simulink model "untitled1"  (R2024b)
settings: Solver=VariableStepAuto  StartTime=0.0  StopTime=10  RelTol=1e-3
values from neighbouring files (symbols this model uses):
  Cd = [0 1]    [mpc3.m]
  Cr = 87342    [mpc3.m]    (also in prueba_mpc.m; prueba_mpc2.m)
  m = 1400    [mpc3.m]    (also in prueba_mpc.m; prueba_mpc2.m)
  R = 1    [prueba_mpc.m]    (also in prueba_mpc2.m)
  vx = 10    [mpc3.m]    (also in prueba_mpc.m; prueba_mpc2.m)
undefined symbols (not defined in the file or in its folder): Af, F_max, FN, g, mode, mu1, mu2, mu3, theta
libraries: slpidlib x1
settings Model: Creator=inaki  LastModifiedBy=inaki
settings DebuggingCC: AlgebraicLoopMsg=none

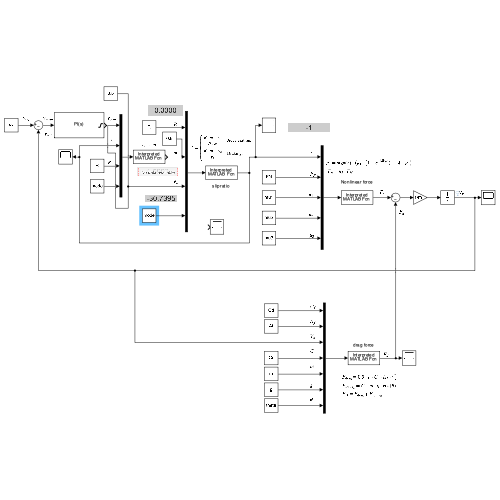
[thumbnail: Simulink's stored preview of the top-level diagram]
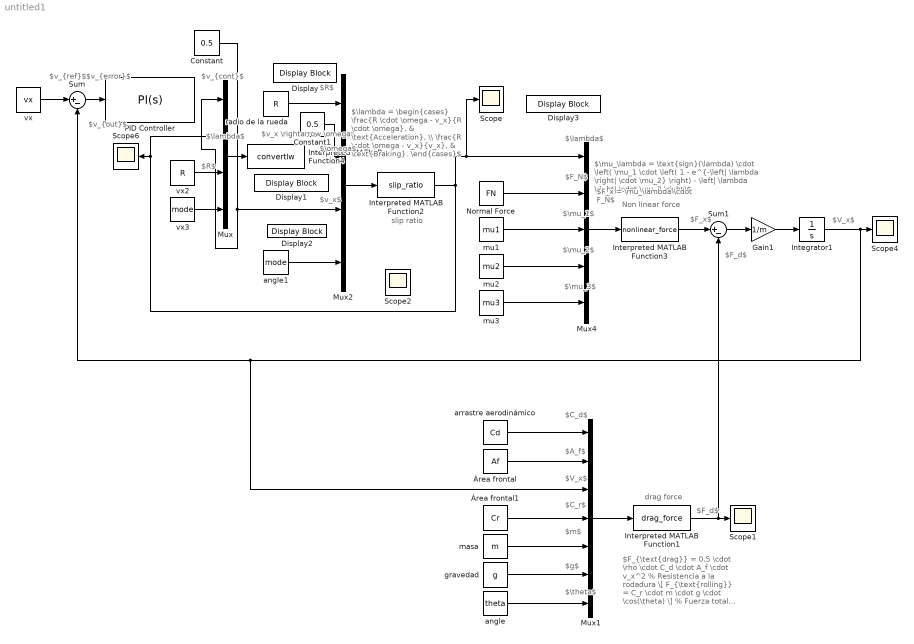
== system untitled1 ==
  note: $R$
  note: $R$
  note: $v_x \rightarrow \omega$
  note: $\mu_\lambda = \text{sign}(\lambda) \cdot \left( \mu_1 \cdot \left( 1 - e^{-\left| \lambda \right| \cdot \mu_2} \right) - \left| \lambda \right| \cdot \mu_3 \right)$
  note: $\mu_3$
  note: $F_x$
  note: $v_x$
  note: $\lambda = \begin{cases} \frac{R \cdot \omega - v_x}{R \cdot \omega}, & \text{Acceleration}, \\ \frac{R \cdot \omega - v_x}{v_x}, & \text{Braking}. \end{cases}$
  note: $\lambda$
  note: $v_{ref}$
  note: $F_d$
  note: $\theta$
  note: $C_d$
  note: Non linear force
  note: $C_r$
  note: slip ratio
  note: $g$
  note: $v_{cont}$
  note: $F_N$
  note: $A_f$
  note: $F_x = \mu_\lambda \cdot F_N$
  note: $\mu_2$
  note: $m$
  note: $\omega$
  note: $F_d$
  note: $\lambda$
  note: $F_{\text{drag}} = 0.5 \cdot \rho \cdot C_d \cdot A_f \cdot v_x^2 % Resistencia a la rodadura \[ F_{\text{rolling}} = C_r \cdot m \cdot g \cdot \cos(\theta) \] % Fuerza total de arrastre \[ F_D = F_{\text{drag}} + F_{\text{rolling}} \]$
  note: $v_{error}$
  note: drag force
  note: $\mu_1$
  note: $V_x$
  note: $V_x$
  note: $v_{out}$
  Constant : Constant  Value=0.5
  Constant1 : Constant  Value=0.5
  Display{,1..3} (4 alike) : DisplayBlock  LabelPosition=Hide  Transparency=1
  Gain1 : Gain  Gain=1/m
  Integrator1 : Integrator
  Interpreted MATLAB Function1 : MATLABFcn  MATLABFcn=drag_force  Output1D=off
  Interpreted MATLAB Function2 : MATLABFcn  MATLABFcn=slip_ratio  Output1D=off
  Interpreted MATLAB Function3 : MATLABFcn  MATLABFcn=nonlinear_force  Output1D=off
  Interpreted MATLAB Function4 : MATLABFcn  MATLABFcn=convertlw  OutputDimensions=1  Output1D=off
  Mux : Mux
  Mux1 : Mux  Inputs=7
  Mux2 : Mux
  Mux4 : Mux  Inputs=5
  Normal Force : Constant  Value=FN
  PID Controller : slpidlib/PID Controller  Controller=PI  Form=Parallel  TimeDomain=Continuous-time  UseExternalTs=off  SampleTime=-1  IntegratorMethod=Forward Euler  FilterMethod=Forward Euler  ControllerParametersSource=internal  P=3371.8  I=1668.7038  UseKiTs=off  D=0  UseExternalDerivativeSource=off  N=100  UseFilter=on  TunerSelectOption=Transfer Function Based (PID Tuner App)  InitialConditionSource=internal  InitialConditionForIntegrator=0  InitialConditionForFilter=0  DifferentiatorICPrevScaledInput=0  ExternalReset=none  TrackingMode=off  Kt=1  LimitOutput=on  SatLimitsSource=internal  UpperSaturationLimit=F_max  LowerSaturationLimit=-F_max  LinearizeAsGain=on  AntiWindupMode=clamping  Kb=1  LimitIntegrator=off  UpperIntegratorSaturationLimit=inf  LowerIntegratorSaturationLimit=-inf  POutMin=[]  POutMax=[]  IOutMin=[]  IOutMax=[]  DOutMin=[]  DOutMax=[]  NOutMin=[]  NOutMax=[]  SumOutMin=[]  SumOutMax=[]  SaturationOutMin=[]  SaturationOutMax=[]  PParamMin=[]  PParamMax=[]  IParamMin=[]  IParamMax=[]  DParamMin=[]  DParamMax=[]  NParamMin=[]  NParamMax=[]  KbParamMin=[]  KbParamMax=[]  KtParamMin=[]  KtParamMax=[]  KbOutMin=[]  KbOutMax=[]  KtOutMin=[]  KtOutMax=[]  IntegratorOutMin=[]  IntegratorOutMax=[]  FilterOutMin=[]  FilterOutMax=[]  SumI1OutMin=[]  SumI1OutMax=[]  SumI2OutMin=[]  SumI2OutMax=[]  SumI3OutMin=[]  SumI3OutMax=[]  SumI4OutMin=[]  SumI4OutMax=[]  SumDOutMin=[]  SumDOutMax=[]  DifferentiatorOutMin=[]  DifferentiatorOutMax=[]  FilterDiffOutCoefMin=[]  FilterDiffOutCoefMax=[]  ReciprocalOutMin=[]  ReciprocalOutMax=[]  SumDenOutMin=[]  SumDenOutMax=[]  SumNumOutMin=[]  SumNumOutMax=[]  DivideOutMin=[]  DivideOutMax=[]  UdiffTsProdOutMin=[]  UdiffTsProdOutMax=[]  NTsProdOutMin=[]  NTsProdOutMax=[]  UintegralTsProdOutMin=[]  UintegralTsProdOutMax=[]  UngainTsProdOutMin=[]  UngainTsProdOutMax=[]  ClampingZeroOutDataTypeStr=Inherit: Inherit via back propagation  ClampingZeroOutMin=[]  ClampingZeroOutMax=[]  FilterDenConstantOutDataTypeStr=Inherit: Inherit via back propagation  FilterDenConstantOutMin=[]  FilterDenConstantOutMax=[]  PCopyOutDataTypeStr=Inherit: Inherit via back propagation  PCopyOutMin=[]  PCopyOutMax=[]  NCopyOutDataTypeStr=Inherit: Inherit via back propagation  NCopyOutMin=[]  NCopyOutMax=[]  IntegratorContinuousStateAttributes=''  IntegratorStateMustResolveToSignalObject=off  IntegratorRTWStateStorageClass=Auto  FilterContinuousStateAttributes=''  FilterStateMustResolveToSignalObject=off  FilterRTWStateStorageClass=Auto  ParallelPVariant=InternalParameters  IdealPVariant=Disabled  IVariant=InternalParameters  DVariant=Disabled  IntegratorVariant=Continuous  SatVariant=Enabled  AWVariant=ContClampingParallel  PCopyVariant=Disabled  TRVariant=Disabled  FdbkBlocksVariant=Forward  IdealPFdbkVariant=Disabled  SatFdbkVariant=Disabled  DerivativeFilterVariant=Disabled  NVariant=Disabled  NCopyVariant=Disabled_SignalSpec  FilterICVariant=Disabled  IntegratorICVariant=InternalICs  ExternalResetVariant=Disabled  TRSumVariant=Passthrough  SumFdbkVariant=Disabled  SumVariant=Sum_PI  TsampFilterVariant=InternalTs  TsampNgainVariant=Passthrough  TsampIntegralVariant=Disabled_SignalSpec  ExternalSaturationOutDataTypeStr=Inherit: Same as second input  DerivativeSourceVariant=Disabled  PreIntVariant=InternalPreInt
  Scope{,1..2,4,6} (5 alike) : Scope
  Sum : Sum  Inputs=|+-
  Sum1 : Sum  Inputs=|+-
  angle : Constant  Value=theta  VectorParams1D=off
  angle1 : Constant  Value=mode
  arrastre aerodinámico : Constant  Value=Cd  VectorParams1D=off
  gravedad : Constant  Value=g  VectorParams1D=off
  masa : Constant  Value=m  VectorParams1D=off
  mu1 : Constant  Value=mu1
  mu2 : Constant  Value=mu2
  mu3 : Constant  Value=mu3
  radio de la rueda : Constant  Value=R  VectorParams1D=off
  vx : Constant  Value=vx  VectorParams1D=off
  vx2 : Constant  Value=R  VectorParams1D=off  SampleTime=R
  vx3 : Constant  Value=mode  VectorParams1D=off  SampleTime=mode
  Área frontal : Constant  Value=Af  VectorParams1D=off
  Área frontal1 : Constant  Value=Cr  VectorParams1D=off
  wires:
  vx/1 -> Sum/1
  mu3/1 -> Mux4/5
  Área frontal/1 -> Mux1/2
  arrastre aerodinámico/1 -> Mux1/1
  Normal Force/1 -> Mux4/2
  vx3/1 -> Mux/4
  gravedad/1 -> Mux1/6
  Sum/1 -> PID Controller/1
  Interpreted MATLAB Function1/1 -> Sum1/2, Scope1/1
  Área frontal1/1 -> Mux1/4
  Mux2/1 -> Interpreted MATLAB Function2/1
  Integrator1/1 -> Mux1/3, Sum/2, Scope4/1
  Mux4/1 -> Interpreted MATLAB Function3/1
  Gain1/1 -> Integrator1/1
  vx2/1 -> Mux/3
  masa/1 -> Mux1/5
  angle1/1 -> Mux2/4
  mu1/1 -> Mux4/3
  Mux/1 -> Interpreted MATLAB Function4/1
  mu2/1 -> Mux4/4
  Interpreted MATLAB Function3/1 -> Sum1/1
  radio de la rueda/1 -> Mux2/1
  Mux1/1 -> Interpreted MATLAB Function1/1
  angle/1 -> Mux1/7
  Sum1/1 -> Gain1/1
  Interpreted MATLAB Function2/1 -> Scope/1, Mux4/1, Mux/2, Scope6/1
  Constant/1 -> Mux2/3, Mux/1
  Constant1/1 -> Mux2/2
